simulink model "practica1"  (R2022a)
settings: Solver=VariableStepAuto  StartTime=0.0  StopTime=10.0  RelTol=1e-3
undefined symbols (not defined in the file or in its folder): none, Rec, SDTV, videoinput
libraries: visionconversions x2, visiontextngfix x2, visionstatistics x1, imaqlib x1, visionsources x1
settings Model: Creator=Juan Pablo  LastModifiedBy=Juan Pablo

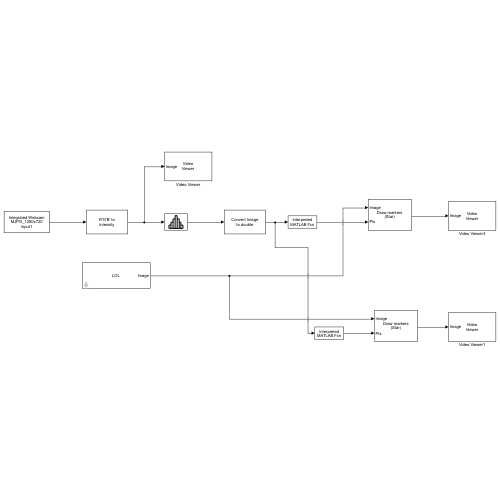
[thumbnail: Simulink's stored preview of the top-level diagram]
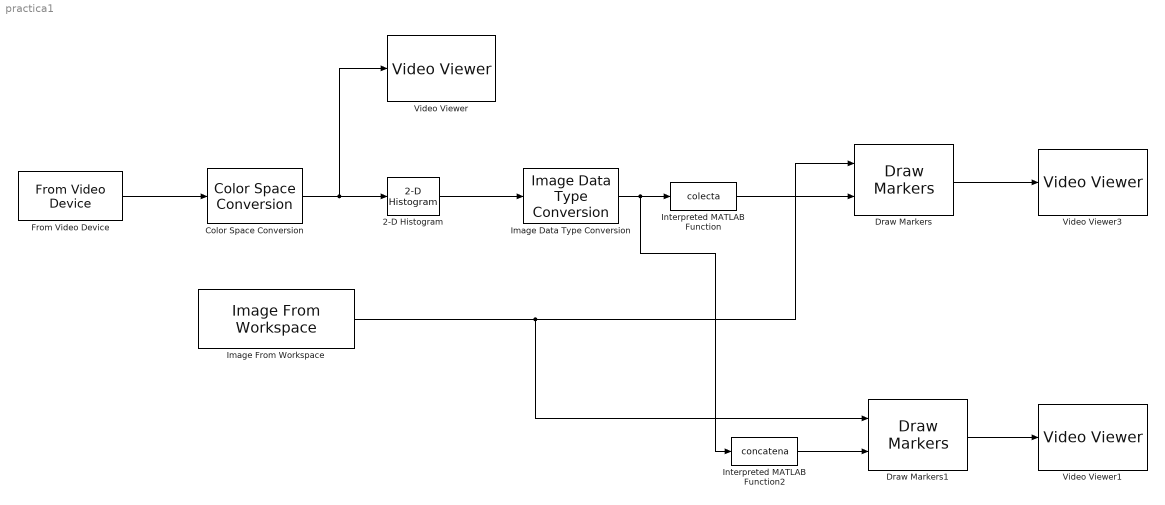
== system practica1 ==
  2-D Histogram : visionstatistics/2-D Histogram  umin=0  umax=1  nbins=256  operateOver=Entire input  normalized=on  run=off  reset=on  trigtype=None  Dimension=1  colComp=on  roundingMode=Floor  overflowMode=off
      settings: SourceProductBaseCode=VP
  Color Space Conversion : visionconversions/Color Space  Conversion  conversion=Obsolete  conversionActive=R'G'B' to intensity  wp_str=D65  rec=Rec. 601 (SDTV)  sys=1125/60/2:1  imagePorts=One multidimensional signal
  Draw Markers : visiontextngfix/Draw Markers  shape=Star  size=3  fill=off  fillClrSource=Specify via dialog  display=Black  intensity=200  color=[200 255 100]  opacity=0.6  viewport=Entire image  antialiasing=off  inType=Obsolete  imagePorts=One multidimensional signal  roundingMode=Floor  overflowMode=off  memoryMode=Specify word length  memoryWordLength=16  memoryFracLength=15  prodOutputMode=Binary point scaling  prodOutputWordLength=32  prodOutputFracLength=14
      settings: SourceProductBaseCode=VP
  Draw Markers1 : visiontextngfix/Draw Markers  shape=Star  size=3  fill=off  fillClrSource=Specify via dialog  display=Black  intensity=200  color=[200 255 100]  opacity=0.6  viewport=Entire image  antialiasing=off  inType=Obsolete  imagePorts=One multidimensional signal  roundingMode=Floor  overflowMode=off  memoryMode=Specify word length  memoryWordLength=16  memoryFracLength=15  prodOutputMode=Binary point scaling  prodOutputWordLength=32  prodOutputFracLength=14
      settings: SourceProductBaseCode=VP
  From Video Device : imaqlib/From Video Device  DeviceMenu=winvideo 1 (Integrated Webcam)  Device=winvideo 1 (Integrated Webcam)  ObjConstructor=videoinput('winvideo', 1)  VideoFormatMenu=MJPG_1280x720  VideoFormat=MJPG_1280x720  VideoSource=input1  ROIPosition=[0 0 720 1280]  EnableHWTrigger=off  TriggerConfiguration=none/none  SampleTime=1/30  OutputPortsMode=One multidimensional signal  DataType=single  CanDoHWTrigger=no  ReturnedColorSpace=rgb  BlockHandle=4.0002  ROIWidth=1280  ROIHeight=720  ROIColumn=0  ROIRow=0  EngXMLPath=C:\Program Files\MATLAB\R2022a\toolbox\imaq\imaq\private  DevXMLPath=C:\ProgramData\MATLAB\SupportPackages\R2022a\toolbox\imaq\supportpackages\genericvideo\adaptor\win64  EngLibPath=C:\Program Files\MATLAB\R2022a\toolbox\imaq\imaqblks\imaqmex\win64  ColorSpace=rgb  BayerSensorAlignment=grbg  ImaqMode=off
  Image Data Type Conversion : visionconversions/Image Data Type Conversion  outDT=double  isSigned=on  wordLen=16  numFracBits=0
      settings: SourceProductBaseCode=VP
  Image From Workspace : visionsources/Image From Workspace  Tag=vipblks_nd  ImageValue=LOL  Ts=inf  imagePorts=One multidimensional signal  OutPortLabels=R|G|B  ImageDataType=Inherit from 'Value'  Signed=on  WordLength=16  sdImageDataType=sfix(16)  FractionLengthMode=User-defined  FractionLength=15
      settings: SourceProductBaseCode=VP
  Interpreted MATLAB Function : MATLABFcn  MATLABFcn=colecta  Output1D=off
  Interpreted MATLAB Function2 : MATLABFcn  MATLABFcn=concatena  Output1D=off
  Video Viewer : VideoViewer  FigPos=[559 583 418 304]
  Video Viewer1 : VideoViewer  FigPos=[187.4 658 417.6 304]
  Video Viewer3 : VideoViewer  FigPos=[890.6 653.2 417.6 304]
  wires:
  From Video Device/1 -> Color Space Conversion/1
  Image Data Type Conversion/1 -> Interpreted MATLAB Function2/1, Interpreted MATLAB Function/1
  Interpreted MATLAB Function/1 -> Draw Markers/2
  Draw Markers/1 -> Video Viewer3/1
  Draw Markers1/1 -> Video Viewer1/1
  Color Space Conversion/1 -> 2-D Histogram/1, Video Viewer/1
  Interpreted MATLAB Function2/1 -> Draw Markers1/2
  2-D Histogram/1 -> Image Data Type Conversion/1
  Image From Workspace/1 -> Draw Markers/1, Draw Markers1/1
